simulink model "blank_canvas_30"  (R2025b)
settings: Solver=FixedStepDiscrete  StartTime=0.0  StopTime=2  FixedStep=Ts  RelTol=1e-3
settings Model: Creator=gdudgeon  LastModifiedBy=gdudgeon
settings DataIOCC: SaveOutput=off  SignalLogging=off  DSMLogging=off  SaveTime=off  ReturnWorkspaceOutputs=off
settings RTWCC: GPUComputeCapability=3.5

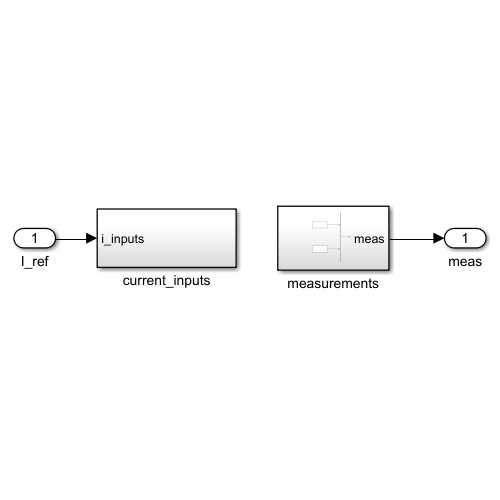
[thumbnail: Simulink's stored preview of the top-level diagram]
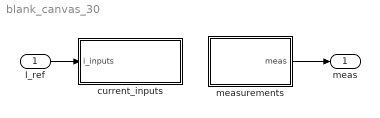
== system blank_canvas_30 ==
  I_ref : Inport
  current_inputs : Subsystem
  measurements : Subsystem
  meas : Outport
  wires:
  measurements/1(meas) -> meas/1
  I_ref/1 -> current_inputs/1(i_inputs)

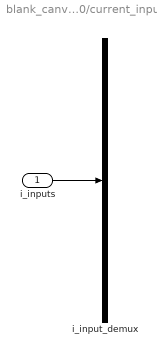
== system blank_canvas_30/current_inputs ==
  i_inputs : Inport
  i_input_demux : Demux  Outputs=2
  wires:
  i_inputs/1 -> i_input_demux/1

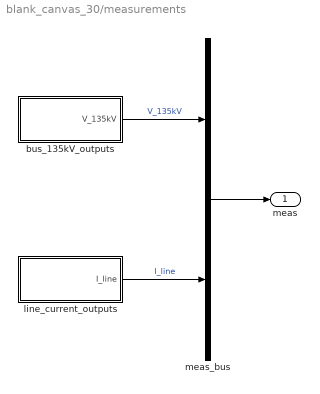
== system blank_canvas_30/measurements ==
  bus_135kV_outputs : Subsystem
  line_current_outputs : Subsystem
  meas_bus : BusCreator  Inputs=2
  meas : Outport
  wires:
  meas_bus/1 -> meas/1
  line_current_outputs/1(I_line) -> meas_bus/2  "I_line"
  bus_135kV_outputs/1(V_135kV) -> meas_bus/1  "V_135kV"

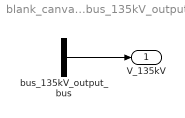
== system blank_canvas_30/measurements/bus_135kV_outputs ==
  bus_135kV_output_bus : BusCreator  Inputs=2
  V_135kV : Outport  VectorParamsAs1DForOutWhenUnconnected=off
  wires:
  bus_135kV_output_bus/1 -> V_135kV/1

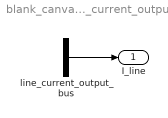
== system blank_canvas_30/measurements/line_current_outputs ==
  line_current_output_bus : BusCreator  Inputs=2
  I_line : Outport  VectorParamsAs1DForOutWhenUnconnected=off
  wires:
  line_current_output_bus/1 -> I_line/1
